simulink library "libMdl_transformVect"  (R2018a)
settings: Solver=VariableStepAuto  StartTime=0.0  StopTime=10.0  RelTol=1e-3
settings Model: Creator=hwinter  LastModifiedBy=Hanno

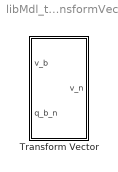
== system libMdl_transformVect ==
  Transform Vector : Subsystem
      mask Display:
      | color('black')
      | port_label('input', 1, 'v^{b}','texmode','on')
      | port_label('input', 2, 'q_b^{n}','texmode','on')
      | port_label('output', 1, 'v^{n}','texmode','on')

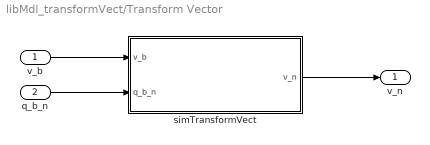
== system libMdl_transformVect/Transform Vector ==
  v_b : Inport
  q_b_n : Inport  Port=2
  simTransformVect : MATLAB Function  TreatAsAtomicUnit=on
  v_n : Outport
  wires:
  simTransformVect/1(v_n) -> v_n/1
  q_b_n/1 -> simTransformVect/2(q_b_n)
  v_b/1 -> simTransformVect/1(v_b)

== matlab function libMdl_transformVect/Transform Vector/simTransformVect ==
  data: v_b input; v_n output; q_b_n input
function v_n = simTransformVect(v_b,q_b_n)

v_n = transformVect(v_b,q_b_n);

end % function
